simulink model "LA_1a"  (R2021a)
settings: Solver=VariableStepAuto  StartTime=0.0  StopTime=10.0  RelTol=1e-3
model workspace (MAT data in the model file):
  G = 5395.5
  T_m = 0.2
  g = 9.81
  k_m = 100
  m = 550
  m_G = 450
libraries: Regler x5
settings Model: OrderedModelArguments=off  Creator=Manoli  LastModifiedBy=Manoli

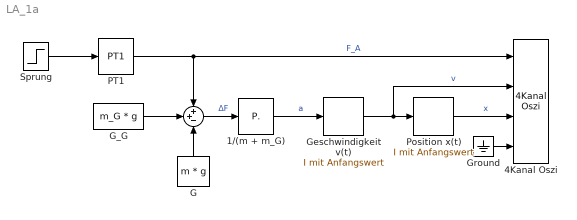
== system LA_1a ==
  " " : Sum  Inputs=++-  InputSameDT=on  SaturateOnIntegerOverflow=on  OutDataTypeStr=Inherit: Same as first input
  1/(m + m_G) : Regler/P.  k=1/(m + m_G)
  4Kanal Oszi : Regler/4Kanal Oszi  N=20000  k=[1 1 1 1]  y=[-5 5]  tmax=1
  G : Constant  Value=m * g
  G_G : Constant  Value=m_G * g
  Geschwindigkeit v(t) : Regler/I mit Anfangswert  Ti=1  u0=0
  Ground : Ground
  PT1 : Regler/PT1  k=k_m  T1=T_m
  Position x(t) : Regler/I mit Anfangswert  Ti=1  u0=10
  Sprung : Step  Time=0.000001  After=0  SampleTime=0
  wires:
  Geschwindigkeit v(t)/1 -> 4Kanal Oszi/2, Position x(t)/1  "v"
  Position x(t)/1 -> 4Kanal Oszi/3  "x"
  " "/1 -> 1/(m + m_G)/1  "ΔF"
  G/1 -> " "/3
  G_G/1 -> " "/2
  Sprung/1 -> PT1/1
  PT1/1 -> 4Kanal Oszi/1, " "/1  "F_A"
  1/(m + m_G)/1 -> Geschwindigkeit v(t)/1  "a"
  Ground/1 -> 4Kanal Oszi/4
